simulink model "SF029A_StabyCmp"  (R2013b)
settings: Solver=FixedStepDiscrete  SolverMode=SingleTasking  StartTime=0.0  StopTime=1  FixedStep=0.002  RelTol=1e-3
values from neighbouring files (symbols this model uses):
  ARCHGLBPRM_2MILLISEC_SEC_F32 = DataDict.Constant    [SF029A_StabyCmp_DataDict.m]
  CMPINPLIM_MOTNWTMTR_F32 = DataDict.Constant    [SF029A_StabyCmp_DataDict.m]
  FLTINJ_STABYCMP_ASSICMD = DataDict.Constant    [SF029A_StabyCmp_DataDict.m]
undefined symbols (not defined in the file): StabyCmpNotchFil1Struct, StabyCmpNotchFil2Struct, StabyCmpNotchFil3Struct, StabyCmpNotchFil4Struct
libraries: NxtrMath x5, FixdToFloat x5, FloatToFixd x5, BilnrIntrpnMplX x4, Fil x2, NxtrLim x2, simulink x1, NxtrAbslt x1, LnrIntrpn x1
(part 1 of 2)
Description:
  | This function provides in-vehicle stability of EPS behavior.  To maximize steering feel, the function blends between two
  |  different tunings based on vehicle speed and low frequency handwheel torque.  Because system gains may get multiplied by various
  |  scale factors, either from serial communications or from other software functions, this function provides a second blending
  |  feature.
  | 
  | Some vehicle programs require a secondary, or "systematic", calculation of stability compensation followed by a correlation check.  The
  | systematic calculations usually must reside in a separate Memory Partition Unit (MPU), and switching between MPUs negatively impacts
  | system throughput.  This model is designed using the best-known implementation at this time.
settings Model: Creator=lzz0tm  LastModifiedBy=XZB1DB
settings Model: ModifiedHistory=|
  | 001
  | Initial release
  | K. Derry
  | n/a
  | 
  | 002
  | WHAT IS THIS ?????????????
  | 
  | 003
  | Move signal summation into SF-34 Assist Firewall.
  | Added AsstFW_Active as new input.
  | K. Derry
  | 19-Apr-2012
  | ICR-3358
  | 
  | 004
  | Addition of LPF of handwheel torque to the compensator blend tables.
  | Changed blend tables from 5x5 to 8x6 (speed x torq)
  | Price Lefler
  | 27-Jun-2012
  | ICR-3562
  | 
  | 005
  | Added functionality to allow compensators 2 and 4 to blend to zero (create two new calibrations)
  | Added 8.8Nm final saturation block to match code. (ref Anomaly 3559)
  | M. Hales
  | 24-Sep-2012
  | ICR-3754
  | Anom-3559
  | 
  | 006
  | Eliminate redundant compensator for BaseAssist input.
  | Eliminate output named BaseAssist_StCmp.
  | Add diverse Systematic Stability Comp.
  | Add correlation check and NTC output signal.
  | Reduce table sizes to 6 vehicle speeds, 5 points each.
  | Eliminate supplemental Word doc.
  | K. Derry
  | 12-Feb-2013
  | ICR-3950
  | 
  | 
  | 007
  | Add Pstep/Nstep counter to Correlation Check.
  | Change verbiage of v006 change log (did not eliminate 3-4 blend table).
  | Add simulation display variable to represent existing code's "StabilityComp2_SysAssistCmd" signal.
  | K. Derry
  | 15-Apr-2013
  | ICR-4078
settings SolverCC: AutoInsertRateTranBlk=on  InsertRTBMode=Always
settings DataIOCC: LimitDataPoints=off  SaveFormat=Structure  ReturnWorkspaceOutputs=on
settings OptimizationCC: BlockReduction=off  InlineParams=on  ZeroExternalMemoryAtStartup=off  ZeroInternalMemoryAtStartup=off  OptimizeModelRefInitCode=on  LifeSpan=1
settings DebuggingCC: ConsistencyChecking=warning  ArrayBoundsChecking=warning  SignalInfNanChecking=error  SignalRangeChecking=warning  UnderspecifiedInitializationDetection=Simplified  SolverPrmCheckMsg=error  InheritedTsInSrcMsg=error  DiscreteInheritContinuousMsg=error  SingleTaskRateTransMsg=error  TasksWithSamePriorityMsg=error  SigSpecEnsureSampleTimeMsg=error  CheckMatrixSingularityMsg=error  ParameterUnderflowMsg=error  ParameterPrecisionLossMsg=error  ParameterTunabilityLossMsg=error  FixptConstUnderflowMsg=warning  FixptConstOverflowMsg=warning  VectorMatrixConversionMsg=error  SignalLabelMismatchMsg=error  UnconnectedInputMsg=error  UnconnectedOutputMsg=error  UnconnectedLineMsg=error  SFcnCompatibilityMsg=error  UniqueDataStoreMsg=warning  BusObjectLabelMismatch=error  RootOutportRequireBusObject=error  AssertControl=DisableAll  ModelReferenceIOMsg=error  ModelReferenceVersionMismatchMessage=warning  ModelReferenceIOMismatchMessage=error  ModelReferenceCSMismatchMessage=warning  ModelReferenceDataLoggingMessage=error  StateNameClashWarn=warning  StrictBusMsg=ErrorOnBusTreatedAsVector  NonBusSignalsTreatedAsBus=error  SFUnexpectedBacktrackingDiag=error  SFInvalidInputDataAccessInChartInitDiag=error  SFNoUnconditionalDefaultTransitionDiag=error  SFTransitionOutsideNaturalParentDiag=error  SFUnconditionalTransitionShadowingDiag=error  SFUndirectedBroadcastEventsDiag=error
settings ModelReferenceCC: ModelReferenceNumInstancesAllowed=Single
settings RTWCC: SystemTargetFile=autosar.tlc  GenCodeOnly=on  TemplateMakefile=ert_default_tmf  Description=AUTOSAR  GenerateReport=on  ProcessScript=autosar_make_rtw_hook  LaunchReport=on
settings CodeAppCC: GenerateComments=off  IgnoreCustomStorageClasses=off  CustomSymbolStrType=$N$R$M  CustomSymbolStrBlkIO=$N$M  SimulinkBlockComments=off
settings STFCustomTargetCC: ParMdlRefBuildCompliant=on  CompOptLevelCompliant=on  IncludeMdlTerminateFcn=off  CombineOutputUpdateFcns=on  SuppressErrorStatus=on  ERTFirstTimeCompliant=on  ERTCustomFileBanners=on  SupportNonFinite=off  SupportComplex=off  SupportContinuousTime=off  SupportNonInlinedSFcns=off  MATLABClassNameForMDSCustomization=Simulink.SoftwareTarget.ERTCustomization  AutosarCompliant=on  GRTInterface=off  SystemTargetFile=autosar.tlc
settings ERTTargetCC: CodeReplacementLibrary=ANSI_C  ConcurrentExecutionCompliant=off  IncludeMdlTerminateFcn=off  SuppressErrorStatus=on  SupportNonFinite=off  SupportComplex=off  ModelStepFunctionPrototypeControlCompliant=off  CPPClassGenCompliant=off  AutosarCompliant=on  InlinedParameterPlacement=NonHierarchical  ERTCustomFileTemplate=example_file_process.tlc  EnableUserReplacementTypes=on

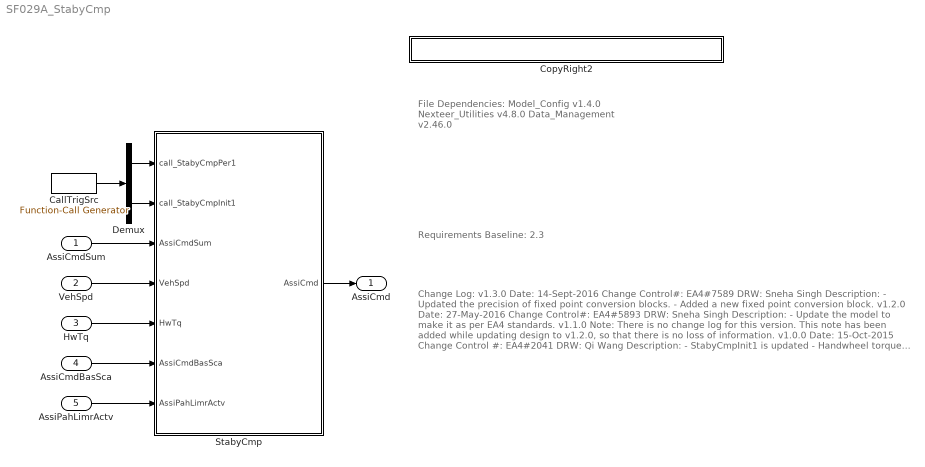
== system SF029A_StabyCmp ==
  note: File Dependencies:
      |
      | Model_Config v1.4.0
      | Nexteer_Utilities v4.8.0
      | Data_Management v2.46.0
  note: Requirements Baseline: 2.3
  note: Change Log:
      |
      | v1.3.0
      | Date: 14-Sept-2016
      | Change Control#: EA4#7589
      | DRW: Sneha Singh
      | Description:
      | - Updated the precision of fixed point conversion blocks.
      | - Added a new fixed point conversion block.
      |
      | v1.2.0
      | Date: 27-May-2016
      | Change Control#: EA4#5893
      | DRW: Sneha Singh
      | Description:
      | - Update the model to make it as per EA4 standards.
      |
      | v1.1.0
      | Note: There is no change log for this version. This note has been
      | added while updating design to v1.2.0, so that there is no loss of
      | information.
      |
      | v1.0.0
      | Date: 15-Oct-2015
      | Change Control #: EA4#2041
      | DRW:  Qi Wang
      | Description:
      | - StabyCmpInit1 is updated
      | - Handwheel torque Low-Pass filter is updated based on 2015 FDD standard
      | - PIMs are updated in the model
  AssiCmdSum : Inport  RequirementInfo="{'linktype_rmi_doors' '0000a537 (/E-STEER Core/SubSystem Specifications/Application Functions/SF029A Stability Compensation)' '#SF029A_70' 'true' 'REQ:  SF029A_70' '' } %GIDa_565dcead_0bc7_40e5_b597_0c44695b6e32"
  VehSpd : Inport  RequirementInfo="{'linktype_rmi_doors' '0000a537 (/E-STEER Core/SubSystem Specifications/Application Functions/SF029A Stability Compensation)' '#SF029A_71' 'true' 'REQ:  SF029A_71' '' } %GIDa_d041abf9_c003_46d5_8c18_c9951e1c5ae1"  Port=2
  HwTq : Inport  RequirementInfo="{'linktype_rmi_doors' '0000a537 (/E-STEER Core/SubSystem Specifications/Application Functions/SF029A Stability Compensation)' '#SF029A_72' 'true' 'REQ:  SF029A_72' '' } %GIDa_dac3164c_f505_4145_8387_4495c6482d18"  Port=3
  AssiCmdBasSca : Inport  RequirementInfo="{'linktype_rmi_doors' '0000a537 (/E-STEER Core/SubSystem Specifications/Application Functions/SF029A Stability Compensation)' '#SF029A_73' 'true' 'REQ:  SF029A_73' '' } %GIDa_6f59ef3f_1a47_4437_bb00_97dd4e07e97c"  Port=4
  AssiPahLimrActv : Inport  RequirementInfo="{'linktype_rmi_doors' '0000a537 (/E-STEER Core/SubSystem Specifications/Application Functions/SF029A Stability Compensation)' '#SF029A_74' 'true' 'REQ:  SF029A_74' '' } %GIDa_e47b1a13_d7c8_4723_b64a_afff46581b7f"  Port=5
  CallTrigSrc : simulink/Ports & Subsystems/Function-Call Generator  RequirementInfo={} %GIDa_050e24ca_7982_42dd_bdc0_09948903a5d2  sample_time=0.004  numberOfIterations=1
  CopyRight2 : Subsystem  Description=|  mask(Copyright Information){none=on}
      | Copyright info block.                                               
      |                                                                     
      | Place copyright information at the top of every subsystem in design.
      mask prompts: none "No parameters"
      mask help: Place copyright information at the top of every subsystem in design.
      mask Display:
      | NxtrConf = 'Nexteer Confidential';
      | 
      | sys = bdroot; %handle for the current model ("system")
      | first = get_param(sys,'Created');
      | if(isempty(first))
      |     first = datestr(now,'yyyy');
      | else
      |     first = first(end-3:end);  %year is last four digits
      | end
      | 
      | last = get_param(sys,'LastModifiedDate');
      | if isempty(last)
      |     last = datestr(now,'yyyy');
      | else
      |     last = last(end-3:end);
      | end
      | 
      | if strcmp(first,last)
      |     fprintf('%s -- Copyright %s Nexteer',NxtrConf,first)
      | else
      |     fprintf('%s -- %s%s- %s Nexteer',NxtrConf,char(169),first,last)
      | end
  Demux : Demux  Outputs=2
  StabyCmp : Subsystem
  AssiCmd : Outport  RequirementInfo="{'linktype_rmi_doors' '0000a537 (/E-STEER Core/SubSystem Specifications/Application Functions/SF029A Stability Compensation)' '#SF029A_76' 'true' 'REQ:  SF029A_76' '' ; 'linktype_rmi_doors' '0000a537 (/E-STEER Core/SubSystem Specifications/Application Functions/SF029A Stability Compensation)' '#SF029A_99' 'true' 'REQ:  SF029A_99' '' ; 'linktype_rmi_doors' '0000a537 (/E-STEER Core/SubSystem Specifications/Application Functions/SF029A Stability Compensation)' '#SF029A_101' 'true' 'REQ:  SF029A_101' '' } %GIDa_32d67de0_2e1d_41c7_bc59_3e04764ffb88"
  wires:
  StabyCmp/1(AssiCmd) -> AssiCmd/1
  AssiCmdSum/1 -> StabyCmp/3(AssiCmdSum)
  VehSpd/1 -> StabyCmp/4(VehSpd)
  HwTq/1 -> StabyCmp/5(HwTq)
  AssiCmdBasSca/1 -> StabyCmp/6(AssiCmdBasSca)
  AssiPahLimrActv/1 -> StabyCmp/7(AssiPahLimrActv)
  Demux/1 -> StabyCmp/1(call_StabyCmpPer1)
  Demux/2 -> StabyCmp/2(call_StabyCmpInit1)
  CallTrigSrc/1 -> Demux/1

== system SF029A_StabyCmp/CopyRight2 ==

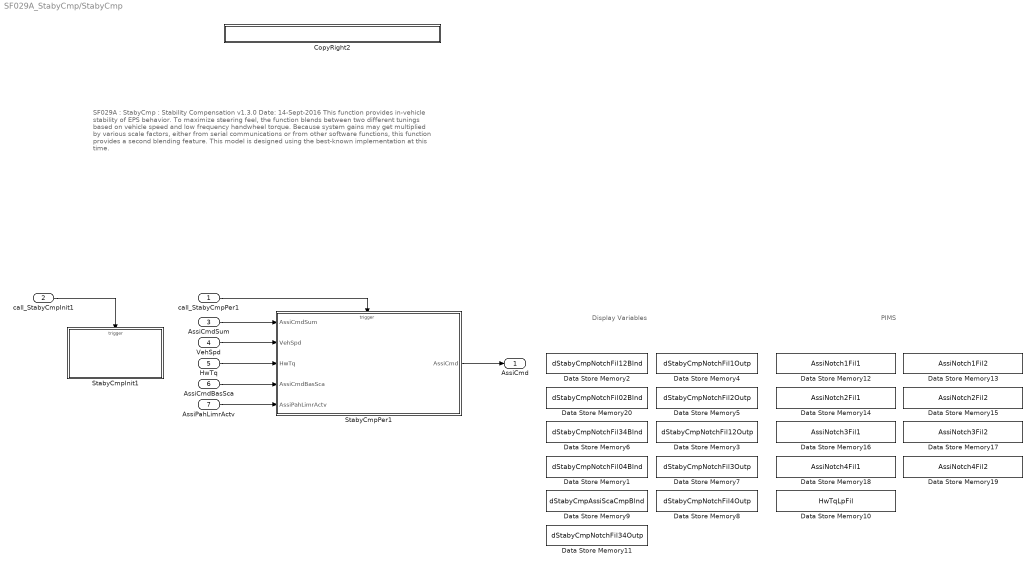
== system SF029A_StabyCmp/StabyCmp ==
  note: SF029A : StabyCmp : Stability Compensation
      | v1.3.0
      | Date: 14-Sept-2016
      |
      |
      |   This function provides in-vehicle stability of EPS behavior. To maximize steering feel,
      |   the function blends between two different tunings based on vehicle speed and low frequency
      |   handwheel torque. Because system gains may get multiplied by various scale factors, either
      |   from serial communications or from other software functions, this function provides a second blending feature.
      |   This model is designed using the best-known implementation at this time.
  note: Display Variables
  note: PIMS
  call_StabyCmpPer1 : Inport
  call_StabyCmpInit1 : Inport  Port=2
  AssiCmdSum : Inport  Port=3
  VehSpd : Inport  Port=4
  HwTq : Inport  Port=5
  AssiCmdBasSca : Inport  Port=6
  AssiPahLimrActv : Inport  Port=7
  CopyRight2 : Subsystem  Description=|  mask(Copyright Information){none=on}
      | Copyright info block.                                               
      |                                                                     
      | Place copyright information at the top of every subsystem in design.
      mask prompts: none "No parameters"
      mask help: Place copyright information at the top of every subsystem in design.
      mask Display:
      | NxtrConf = 'Nexteer Confidential';
      | 
      | sys = bdroot; %handle for the current model ("system")
      | first = get_param(sys,'Created');
      | if(isempty(first))
      |     first = datestr(now,'yyyy');
      | else
      |     first = first(end-3:end);  %year is last four digits
      | end
      | 
      | last = get_param(sys,'LastModifiedDate');
      | if isempty(last)
      |     last = datestr(now,'yyyy');
      | else
      |     last = last(end-3:end);
      | end
      | 
      | if strcmp(first,last)
      |     fprintf('%s -- Copyright %s Nexteer',NxtrConf,first)
      | else
      |     fprintf('%s -- %s%s- %s Nexteer',NxtrConf,char(169),first,last)
      | end
  Data Store Memory1 : DataStoreMemory  DataStoreName=dStabyCmpNotchFil04Blnd  ReadBeforeWriteMsg=warning  WriteAfterWriteMsg=warning  WriteAfterReadMsg=warning  StateMustResolveToSignalObject=on
  Data Store Memory10 : DataStoreMemory  DataStoreName=HwTqLpFil  InitialValue=[]  StateMustResolveToSignalObject=on
  Data Store Memory11 : DataStoreMemory  DataStoreName=dStabyCmpNotchFil34Outp  ReadBeforeWriteMsg=warning  WriteAfterWriteMsg=warning  WriteAfterReadMsg=warning  StateMustResolveToSignalObject=on
  Data Store Memory12 : DataStoreMemory  DataStoreName=AssiNotch1Fil1  StateMustResolveToSignalObject=on
  Data Store Memory13 : DataStoreMemory  DataStoreName=AssiNotch1Fil2  InitialValue=[]  StateMustResolveToSignalObject=on
  Data Store Memory14 : DataStoreMemory  DataStoreName=AssiNotch2Fil1  InitialValue=[]  StateMustResolveToSignalObject=on
  Data Store Memory15 : DataStoreMemory  DataStoreName=AssiNotch2Fil2  InitialValue=[]  StateMustResolveToSignalObject=on
  Data Store Memory16 : DataStoreMemory  DataStoreName=AssiNotch3Fil1  InitialValue=[]  StateMustResolveToSignalObject=on
  Data Store Memory17 : DataStoreMemory  DataStoreName=AssiNotch3Fil2  InitialValue=[]  StateMustResolveToSignalObject=on
  Data Store Memory18 : DataStoreMemory  DataStoreName=AssiNotch4Fil1  InitialValue=[]  StateMustResolveToSignalObject=on
  Data Store Memory19 : DataStoreMemory  DataStoreName=AssiNotch4Fil2  InitialValue=[]  StateMustResolveToSignalObject=on
  Data Store Memory2 : DataStoreMemory  DataStoreName=dStabyCmpNotchFil12Blnd  ReadBeforeWriteMsg=warning  WriteAfterWriteMsg=warning  WriteAfterReadMsg=warning  StateMustResolveToSignalObject=on
  Data Store Memory20 : DataStoreMemory  DataStoreName=dStabyCmpNotchFil02Blnd  ReadBeforeWriteMsg=warning  WriteAfterWriteMsg=warning  WriteAfterReadMsg=warning  StateMustResolveToSignalObject=on
  Data Store Memory3 : DataStoreMemory  DataStoreName=dStabyCmpNotchFil12Outp  ReadBeforeWriteMsg=warning  WriteAfterWriteMsg=warning  WriteAfterReadMsg=warning  StateMustResolveToSignalObject=on
  Data Store Memory4 : DataStoreMemory  DataStoreName=dStabyCmpNotchFil1Outp  ReadBeforeWriteMsg=warning  WriteAfterWriteMsg=warning  WriteAfterReadMsg=warning  StateMustResolveToSignalObject=on
  Data Store Memory5 : DataStoreMemory  DataStoreName=dStabyCmpNotchFil2Outp  ReadBeforeWriteMsg=warning  WriteAfterWriteMsg=warning  WriteAfterReadMsg=warning  StateMustResolveToSignalObject=on
  Data Store Memory6 : DataStoreMemory  DataStoreName=dStabyCmpNotchFil34Blnd  ReadBeforeWriteMsg=warning  WriteAfterWriteMsg=warning  WriteAfterReadMsg=warning  StateMustResolveToSignalObject=on
  Data Store Memory7 : DataStoreMemory  DataStoreName=dStabyCmpNotchFil3Outp  ReadBeforeWriteMsg=warning  WriteAfterWriteMsg=warning  WriteAfterReadMsg=warning  StateMustResolveToSignalObject=on
  Data Store Memory8 : DataStoreMemory  DataStoreName=dStabyCmpNotchFil4Outp  ReadBeforeWriteMsg=warning  WriteAfterWriteMsg=warning  WriteAfterReadMsg=warning  StateMustResolveToSignalObject=on
  Data Store Memory9 : DataStoreMemory  DataStoreName=dStabyCmpAssiScaCmpBlnd  ReadBeforeWriteMsg=warning  WriteAfterWriteMsg=warning  WriteAfterReadMsg=warning  StateMustResolveToSignalObject=on
  StabyCmpInit1 : Subsystem
  StabyCmpPer1 : Subsystem
  AssiCmd : Outport
  wires:
  AssiCmdSum/1 -> StabyCmpPer1/1(AssiCmdSum)
  VehSpd/1 -> StabyCmpPer1/2(VehSpd)
  HwTq/1 -> StabyCmpPer1/3(HwTq)
  AssiCmdBasSca/1 -> StabyCmpPer1/4(AssiCmdBasSca)
  AssiPahLimrActv/1 -> StabyCmpPer1/5(AssiPahLimrActv)
  StabyCmpPer1/1(AssiCmd) -> AssiCmd/1
  call_StabyCmpPer1/1 -> StabyCmpPer1/Trigger
  call_StabyCmpInit1/1 -> StabyCmpInit1/Trigger

== system SF029A_StabyCmp/StabyCmp/CopyRight2 ==

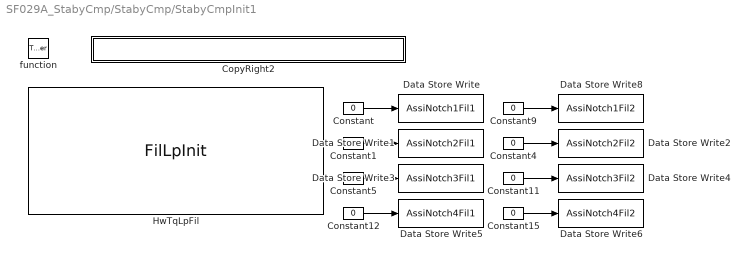
== system SF029A_StabyCmp/StabyCmp/StabyCmpInit1 ==
  function : TriggerPort  TriggerType=function-call
  Constant{,1,4..5,9,11..12,15} (8 alike) : Constant  Value=0  OutDataTypeStr=Inherit: Inherit via back propagation  SampleTime=-1
  CopyRight2 : Subsystem  Description=|  mask(Copyright Information){none=on}
      | Copyright info block.                                               
      |                                                                     
      | Place copyright information at the top of every subsystem in design.
      mask prompts: none "No parameters"
      mask help: Place copyright information at the top of every subsystem in design.
      mask Display:
      | NxtrConf = 'Nexteer Confidential';
      | 
      | sys = bdroot; %handle for the current model ("system")
      | first = get_param(sys,'Created');
      | if(isempty(first))
      |     first = datestr(now,'yyyy');
      | else
      |     first = first(end-3:end);  %year is last four digits
      | end
      | 
      | last = get_param(sys,'LastModifiedDate');
      | if isempty(last)
      |     last = datestr(now,'yyyy');
      | else
      |     last = last(end-3:end);
      | end
      | 
      | if strcmp(first,last)
      |     fprintf('%s -- Copyright %s Nexteer',NxtrConf,first)
      | else
      |     fprintf('%s -- %s%s- %s Nexteer',NxtrConf,char(169),first,last)
      | end
  Data Store Write : DataStoreWrite  DataStoreName=AssiNotch1Fil1  DataStoreElements=AssiNotch1Fil1
  Data Store Write1 : DataStoreWrite  DataStoreName=AssiNotch2Fil1  DataStoreElements=AssiNotch2Fil1
  Data Store Write2 : DataStoreWrite  DataStoreName=AssiNotch2Fil2  DataStoreElements=AssiNotch2Fil2
  Data Store Write3 : DataStoreWrite  DataStoreName=AssiNotch3Fil1  DataStoreElements=AssiNotch3Fil1
  Data Store Write4 : DataStoreWrite  DataStoreName=AssiNotch3Fil2  DataStoreElements=AssiNotch3Fil2
  Data Store Write5 : DataStoreWrite  DataStoreName=AssiNotch4Fil1  DataStoreElements=AssiNotch4Fil1
  Data Store Write6 : DataStoreWrite  DataStoreName=AssiNotch4Fil2  DataStoreElements=AssiNotch4Fil2
  Data Store Write8 : DataStoreWrite  DataStoreName=AssiNotch1Fil2  DataStoreElements=AssiNotch1Fil2
  HwTqLpFil : Fil/FilLpInit  Ic=0  Ts=ARCHGLBPRM_2MILLISEC_SEC_F32  Freq=StabyCmpHwTqLpFilFrq  StVar=HwTqLpFil
  wires:
  Constant/1 -> Data Store Write/1
  Constant9/1 -> Data Store Write8/1
  Constant1/1 -> Data Store Write1/1
  Constant4/1 -> Data Store Write2/1
  Constant5/1 -> Data Store Write3/1
  Constant11/1 -> Data Store Write4/1
  Constant12/1 -> Data Store Write5/1
  Constant15/1 -> Data Store Write6/1

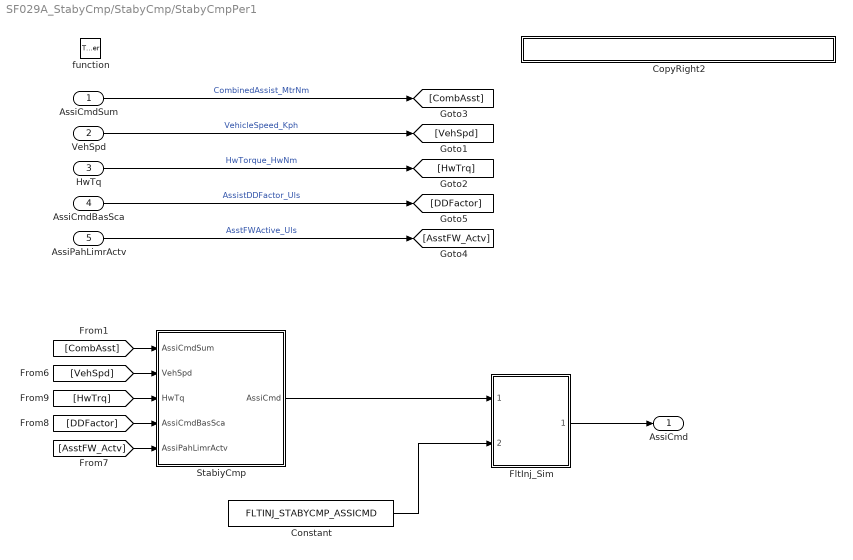
== system SF029A_StabyCmp/StabyCmp/StabyCmpPer1 ==
  AssiCmdSum : Inport
  VehSpd : Inport  Port=2
  HwTq : Inport  Port=3
  AssiCmdBasSca : Inport  Port=4
  AssiPahLimrActv : Inport  Port=5
  function : TriggerPort  TriggerType=function-call  PortDimensions=1
  Constant : Constant  Value=FLTINJ_STABYCMP_ASSICMD
  CopyRight2 : Subsystem  Description=|  mask(Copyright Information){none=on}
      | Copyright info block.                                               
      |                                                                     
      | Place copyright information at the top of every subsystem in design.
      mask prompts: none "No parameters"
      mask help: Place copyright information at the top of every subsystem in design.
      mask Display:
      | NxtrConf = 'Nexteer Confidential';
      | 
      | sys = bdroot; %handle for the current model ("system")
      | first = get_param(sys,'Created');
      | if(isempty(first))
      |     first = datestr(now,'yyyy');
      | else
      |     first = first(end-3:end);  %year is last four digits
      | end
      | 
      | last = get_param(sys,'LastModifiedDate');
      | if isempty(last)
      |     last = datestr(now,'yyyy');
      | else
      |     last = last(end-3:end);
      | end
      | 
      | if strcmp(first,last)
      |     fprintf('%s -- Copyright %s Nexteer',NxtrConf,first)
      | else
      |     fprintf('%s -- %s%s- %s Nexteer',NxtrConf,char(169),first,last)
      | end
  FltInj_Sim : Subsystem  RequirementInfo="{'linktype_rmi_doors' '0000a537 (/E-STEER Core/SubSystem Specifications/Application Functions/SF029A Stability Compensation)' '#SF029A_106' 'true' 'REQ:  SF029A_106' '' } %GIDa_4f586a3b_dea5_4a76_a847_596b049200d7"  TreatAsAtomicUnit=on  VariantControl=FltInj_sim  mask(Fault_Injection){}
      mask help: Fault Injection is a simulation only block for EA3 and EA4 programs.
  StabiyCmp : Subsystem
  AssiCmd : Outport
  wires:
  VehSpd/1 -> [VehSpd]  "VehicleSpeed_Kph"
  HwTq/1 -> [HwTrq]  "HwTorque_HwNm"
  [CombAsst] -> StabiyCmp/1(AssiCmdSum)
  [VehSpd] -> StabiyCmp/2(VehSpd)
  [HwTrq] -> StabiyCmp/3(HwTq)
  [DDFactor] -> StabiyCmp/4(AssiCmdBasSca)
  AssiCmdSum/1 -> [CombAsst]  "CombinedAssist_MtrNm"
  AssiCmdBasSca/1 -> [DDFactor]  "AssistDDFactor_Uls"
  AssiPahLimrActv/1 -> [AsstFW_Actv]  "AsstFWActive_Uls"
  [AsstFW_Actv] -> StabiyCmp/5(AssiPahLimrActv)
  Constant/1 -> FltInj_Sim/2(FltInjCon)
  FltInj_Sim/1(AssiCmd) -> AssiCmd/1
  StabiyCmp/1(AssiCmd) -> FltInj_Sim/1(AssiCmdOutp)

== system SF029A_StabyCmp/StabyCmp/StabyCmpInit1/CopyRight2 ==

== system SF029A_StabyCmp/StabyCmp/StabyCmpPer1/CopyRight2 ==

== system SF029A_StabyCmp/StabyCmp/StabyCmpPer1/FltInj_Sim ==
  note: This block requires no modification by FDD author.
      |
      | This block does not actually simulate any fault injection.  It is simply a pass-thru.
      |
      | The port (#2) simply terminates its signal, but we are trying to force the FDD author
      | to properly use the Constant in FDD model.
  note: EA4.x Fault Injection
  note: Inport #2 must be Constant
  AssiCmdOutp : Inport
  FltInjCon : Inport  Port=2
  CopyRight2 : Subsystem  Description=|  mask(Copyright Information){none=on}
      | Copyright info block.                                               
      |                                                                     
      | Place copyright information at the top of every subsystem in design.
      mask prompts: none "No parameters"
      mask help: Place copyright information at the top of every subsystem in design.
      mask Display:
      | NxtrConf = 'Nexteer Confidential';
      | 
      | sys = bdroot; %handle for the current model ("system")
      | first = get_param(sys,'Created');
      | if(isempty(first))
      |     first = datestr(now,'yyyy');
      | else
      |     first = first(end-3:end);  %year is last four digits
      | end
      | 
      | last = get_param(sys,'LastModifiedDate');
      | if isempty(last)
      |     last = datestr(now,'yyyy');
      | else
      |     last = last(end-3:end);
      | end
      | 
      | if strcmp(first,last)
      |     fprintf('%s -- Copyright %s Nexteer',NxtrConf,first)
      | else
      |     fprintf('%s -- %s%s- %s Nexteer',NxtrConf,char(169),first,last)
      | end
  Terminator : Terminator
  AssiCmd : Outport
  wires:
  AssiCmdOutp/1 -> AssiCmd/1
  FltInjCon/1 -> Terminator/1

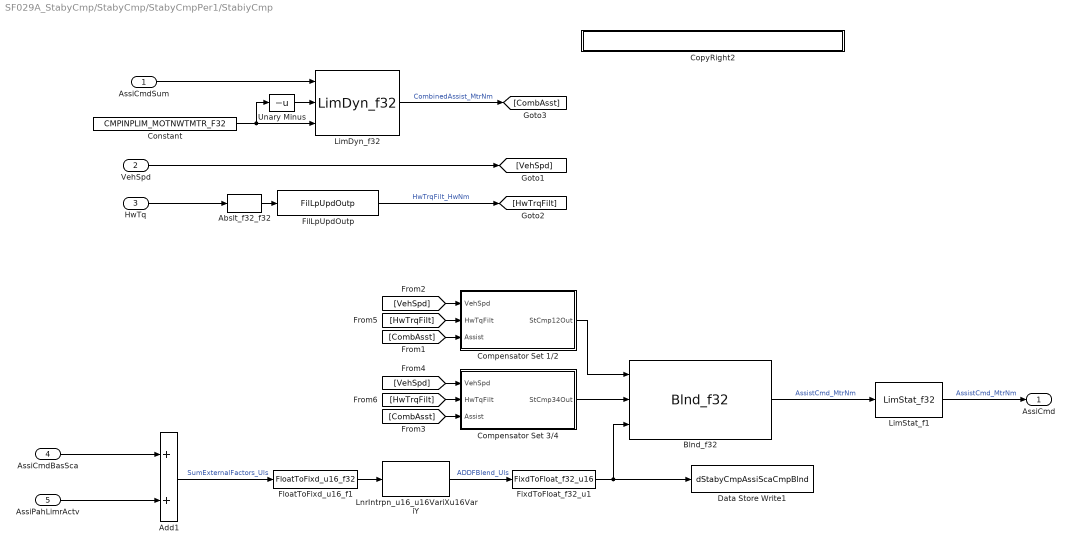
== system SF029A_StabyCmp/StabyCmp/StabyCmpPer1/StabiyCmp ==
  AssiCmdSum : Inport
  VehSpd : Inport  Port=2
  HwTq : Inport  Port=3
  AssiCmdBasSca : Inport  RequirementInfo="{'linktype_rmi_doors' '0000a537 (/E-STEER Core/SubSystem Specifications/Application Functions/SF029A Stability Compensation)' '#SF029A_93' 'true' 'REQ:  SF029A_93' '' } %GIDa_e52f2ad1_fd47_421d_8c08_8c30a1c05406"  Port=4
      settings: AttributesFormatString=%<Tag>
  AssiPahLimrActv : Inport  RequirementInfo="{'linktype_rmi_doors' '0000a537 (/E-STEER Core/SubSystem Specifications/Application Functions/SF029A Stability Compensation)' '#SF029A_93' 'true' 'REQ:  SF029A_93' '' } %GIDa_1d5b88ab_396b_4d89_9700_00f5ed32e8aa"  Port=5
      settings: AttributesFormatString=%<Tag>
  Abslt_f32_f32 : NxtrAbslt/Abslt_f32_f32  RequirementInfo="{'linktype_rmi_doors' '0000a537 (/E-STEER Core/SubSystem Specifications/Application Functions/SF029A Stability Compensation)' '#SF029A_80' 'true' 'REQ:  SF029A_80' '' } %GIDa_e58e449f_99f0_42c1_896c_b4bed6e53470"  SFunctionSpec=single y1 = Abslt_f32_f32(single u1)
      settings: AttributesFormatString=%<Name>
  Add1 : Sum  RequirementInfo="{'linktype_rmi_doors' '0000a537 (/E-STEER Core/SubSystem Specifications/Application Functions/SF029A Stability Compensation)' '#SF029A_93' 'true' 'REQ:  SF029A_93' '' } %GIDa_2f792d03_7f63_496e_bb4b_c1c151e55f4e"
      settings: AttributesFormatString=%<Tag>
  Blnd_f32 : NxtrMath/Blnd_f32  RequirementInfo="{'linktype_rmi_doors' '0000a537 (/E-STEER Core/SubSystem Specifications/Application Functions/SF029A Stability Compensation)' '#SF029A_93' 'true' 'REQ:  SF029A_93' '' } %GIDa_aac33a22_20b9_4488_865f_8251dad173fa"  SFunctionSpec=single y1 = Blnd_f32(single u1, single u2, single u3)  Parameter3=on
      settings: AttributesFormatString=%<Name>
  Compensator Set 1/2 : Subsystem
  Compensator Set 3/4 : Subsystem
  Constant : Constant  RequirementInfo="{'linktype_rmi_doors' '0000a537 (/E-STEER Core/SubSystem Specifications/Application Functions/SF029A Stability Compensation)' '#SF029A_81' 'true' 'REQ:  SF029A_81' '' } %GIDa_0fa329a0_f831_46cf_b20c_4e9a4dd8937d"  Value=CMPINPLIM_MOTNWTMTR_F32
  CopyRight2 : Subsystem  Description=|  mask(Copyright Information){none=on}
      | Copyright info block.                                               
      |                                                                     
      | Place copyright information at the top of every subsystem in design.
      mask prompts: none "No parameters"
      mask help: Place copyright information at the top of every subsystem in design.
      mask Display:
      | NxtrConf = 'Nexteer Confidential';
      | 
      | sys = bdroot; %handle for the current model ("system")
      | first = get_param(sys,'Created');
      | if(isempty(first))
      |     first = datestr(now,'yyyy');
      | else
      |     first = first(end-3:end);  %year is last four digits
      | end
      | 
      | last = get_param(sys,'LastModifiedDate');
      | if isempty(last)
      |     last = datestr(now,'yyyy');
      | else
      |     last = last(end-3:end);
      | end
      | 
      | if strcmp(first,last)
      |     fprintf('%s -- Copyright %s Nexteer',NxtrConf,first)
      | else
      |     fprintf('%s -- %s%s- %s Nexteer',NxtrConf,char(169),first,last)
      | end
  Data Store Write1 : DataStoreWrite  DataStoreName=dStabyCmpAssiScaCmpBlnd
  FilLpUpdOutp : Fil/FilLpUpdOutp  RequirementInfo="{'linktype_rmi_doors' '0000a537 (/E-STEER Core/SubSystem Specifications/Application Functions/SF029A Stability Compensation)' '#SF029A_80' 'true' 'REQ:  SF029A_80' '' } %GIDa_e50dfd97_808a_4ecb_9afb_8d1ce7d9c01b"  StVar=HwTqLpFil
      settings: AttributesFormatString=StVar: %<StVar>
  FixdToFloat_f32_u1 : FixdToFloat/FixdToFloat_f32_u16  RequirementInfo="{'linktype_rmi_doors' '0000a537 (/E-STEER Core/SubSystem Specifications/Application Functions/SF029A Stability Compensation)' '#SF029A_93' 'true' 'REQ:  SF029A_93' '' } %GIDa_8db98107_d72d_46ce_bb11_b21278a91118"  Param1=14
  FloatToFixd_u16_f1 : FloatToFixd/FloatToFixd_u16_f32  Param1=14
  LimDyn_f32 : NxtrLim/LimDyn_f32  RequirementInfo="{'linktype_rmi_doors' '0000a537 (/E-STEER Core/SubSystem Specifications/Application Functions/SF029A Stability Compensation)' '#SF029A_81' 'true' 'REQ:  SF029A_81' '' } %GIDa_138aed1d_98dc_4852_adea_0252395672f7"
  LimStat_f1 : NxtrLim/LimStat_f32  RequirementInfo="{'linktype_rmi_doors' '0000a537 (/E-STEER Core/SubSystem Specifications/Application Functions/SF029A Stability Compensation)' '#SF029A_94' 'true' 'REQ:  SF029A_94' '' } %GIDa_e5042578_7661_4cd7_b5a9_512a3779a978"  LoLim=SYSGLBPRM_MOTTQCMDLOLIM_MOTNWTMTR_F32  HiLim=SYSGLBPRM_MOTTQCMDHILIM_MOTNWTMTR_F32
      settings: AttributesFormatString=|
      | Low Limit: %<LoLim>
      | High Limit:%<HiLim>
  LnrIntrpn_u16_u16VariXu16VariY : LnrIntrpn/LnrIntrpn_u16_u16VariXu16VariY  RequirementInfo="{'linktype_rmi_doors' '0000a537 (/E-STEER Core/SubSystem Specifications/Application Functions/SF029A Stability Compensation)' '#SF029A_93' 'true' 'REQ:  SF029A_93' '' } %GIDa_788cf387_8266_4e90_8950_327c02d399c2"  XTbl=StabyCmpAssiScaBlndX  YTbl=StabyCmpAssiScaBlndY
      settings: AttributesFormatString=|
      | Lnr ( u16VariX , u16VariY )
      | XTbl: %<XTbl>
      | YTbl: %<YTbl>
  Unary Minus : UnaryMinus  RequirementInfo="{'linktype_rmi_doors' '0000a537 (/E-STEER Core/SubSystem Specifications/Application Functions/SF029A Stability Compensation)' '#SF029A_81' 'true' 'REQ:  SF029A_81' '' } %GIDa_4787fd09_3b48_441a_baf7_bf2ffd79fe3e"
  AssiCmd : Outport
  wires:
  Compensator Set 3/4/1(StCmp34Out) -> Blnd_f32/2
  Compensator Set 1/2/1(StCmp12Out) -> Blnd_f32/1
  Blnd_f32/1 -> LimStat_f1/1  "AssistCmd_MtrNm"
  VehSpd/1 -> [VehSpd]
  AssiCmdSum/1 -> LimDyn_f32/1
  Add1/1 -> FloatToFixd_u16_f1/1  "SumExternalFactors_Uls"
  LnrIntrpn_u16_u16VariXu16VariY/1 -> FixdToFloat_f32_u1/1  "ADDFBlend_Uls"
  AssiCmdBasSca/1 -> Add1/1
  AssiPahLimrActv/1 -> Add1/2
  LimDyn_f32/1 -> [CombAsst]  "CombinedAssist_MtrNm"
  LimStat_f1/1 -> AssiCmd/1  "AssistCmd_MtrNm"
  [VehSpd] -> Compensator Set 1/2/1(VehSpd)
  [CombAsst] -> Compensator Set 1/2/3(Assist)
  Abslt_f32_f32/1 -> FilLpUpdOutp/1
  HwTq/1 -> Abslt_f32_f32/1
  FilLpUpdOutp/1 -> [HwTrqFilt]  "HwTrqFilt_HwNm"
  [HwTrqFilt] -> Compensator Set 1/2/2(HwTqFilt)
  [VehSpd] -> Compensator Set 3/4/1(VehSpd)
  [HwTrqFilt] -> Compensator Set 3/4/2(HwTqFilt)
  [CombAsst] -> Compensator Set 3/4/3(Assist)
  FixdToFloat_f32_u1/1 -> Blnd_f32/3, Data Store Write1/1
  Constant/1 -> Unary Minus/1, LimDyn_f32/3
  Unary Minus/1 -> LimDyn_f32/2
  FloatToFixd_u16_f1/1 -> LnrIntrpn_u16_u16VariXu16VariY/1

== system SF029A_StabyCmp/StabyCmp/StabyCmpPer1/FltInj_Sim/CopyRight2 ==

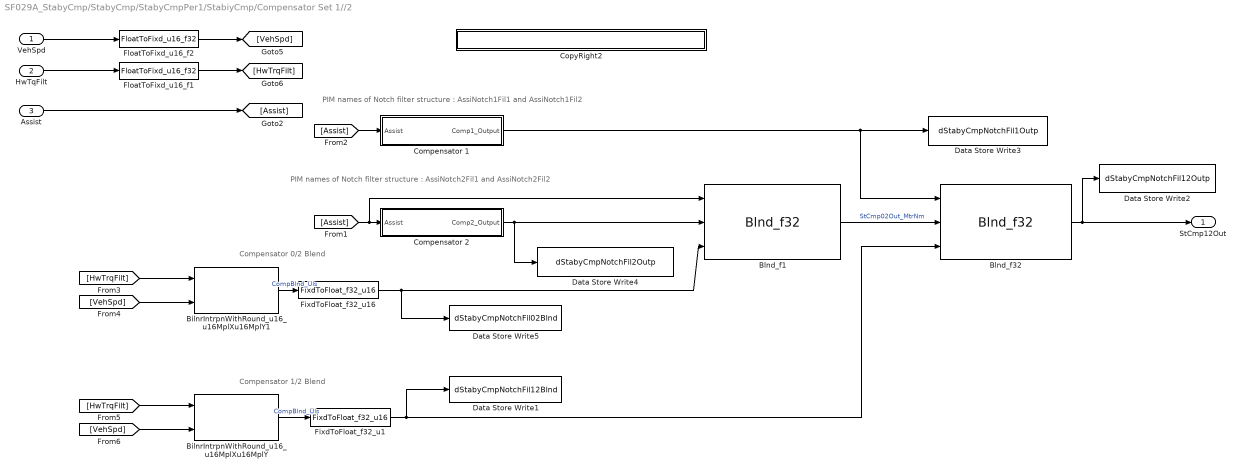
== system SF029A_StabyCmp/StabyCmp/StabyCmpPer1/StabiyCmp/Compensator Set 1//2 ==
  note: PIM names of Notch filter structure : AssiNotch1Fil1 and AssiNotch1Fil2
  note: Compensator 1/2 Blend
  note: Compensator 0/2 Blend
  note: PIM names of Notch filter structure : AssiNotch2Fil1 and AssiNotch2Fil2
  VehSpd : Inport
  HwTqFilt : Inport  Port=2
  Assist : Inport  Port=3
  BilnrIntrpnWithRound_u16_u16MplXu16MplY : BilnrIntrpnMplX/BilnrIntrpnWithRound_u16_u16MplXu16MplY  RequirementInfo="{'linktype_rmi_doors' '0000a537 (/E-STEER Core/SubSystem Specifications/Application Functions/SF029A Stability Compensation)' '#SF029A_86' 'true' 'REQ:  SF029A_86' '' } %GIDa_fadd72e6_d831_45ef_8099_953e3d2c1c69"  MplXTbl=StabyCmpNotchFilBlnd12TqX  MplYTbl=StabyCmpNotchFilBlnd12Y  BilnrSelnTbl=StabyCmpNotchFilBilnrBlndVehSpd
      settings: AttributesFormatString=|
      | Bilnr ( u16MplX , u16MplY )
      | XTbl: %<MplXTbl>
      | YTbl: %<MplYTbl>
      | BilnrSelnTbl: %<BilnrSelnTbl>
  BilnrIntrpnWithRound_u16_u16MplXu16MplY1 : BilnrIntrpnMplX/BilnrIntrpnWithRound_u16_u16MplXu16MplY  RequirementInfo="{'linktype_rmi_doors' '0000a537 (/E-STEER Core/SubSystem Specifications/Application Functions/SF029A Stability Compensation)' '#SF029A_85' 'true' 'REQ:  SF029A_85' '' } %GIDa_42ed8477_37e6_4b44_a66a_f9bae03e7c36"  MplXTbl=StabyCmpNotchFilBlnd12TqX  MplYTbl=StabyCmpNotchFilBlnd02Y  BilnrSelnTbl=StabyCmpNotchFilBilnrBlndVehSpd
      settings: AttributesFormatString=|
      | Bilnr ( u16MplX , u16MplY )
      | XTbl: %<MplXTbl>
      | YTbl: %<MplYTbl>
      | BilnrSelnTbl: %<BilnrSelnTbl>
  Blnd_f1 : NxtrMath/Blnd_f32  RequirementInfo="{'linktype_rmi_doors' '0000a537 (/E-STEER Core/SubSystem Specifications/Application Functions/SF029A Stability Compensation)' '#SF029A_85' 'true' 'REQ:  SF029A_85' '' } %GIDa_dba1abdf_517a_44f0_a412_df1ce507f594"  SFunctionSpec=single y1 = Blnd_f32(single u1, single u2, single u3)  Parameter3=on
      settings: AttributesFormatString=%<Name>
  Blnd_f32 : NxtrMath/Blnd_f32  RequirementInfo="{'linktype_rmi_doors' '0000a537 (/E-STEER Core/SubSystem Specifications/Application Functions/SF029A Stability Compensation)' '#SF029A_86' 'true' 'REQ:  SF029A_86' '' } %GIDa_db82eb3d_baf5_47e3_9dad_3db9927823cc"  SFunctionSpec=single y1 = Blnd_f32(single u1, single u2, single u3)  Parameter3=on
      settings: AttributesFormatString=%<Name>
  Compensator 1 : Subsystem  RequirementInfo="{'linktype_rmi_doors' '0000a537 (/E-STEER Core/SubSystem Specifications/Application Functions/SF029A Stability Compensation)' '#SF029A_84' 'true' 'REQ:  SF029A_84' '' ; 'linktype_rmi_doors' '0000a537 (/E-STEER Core/SubSystem Specifications/Application Functions/SF029A Stability Compensation)' '#SF029A_86' 'true' 'REQ:  SF029A_86' '' } %GIDa_51cc23fa_f620_4c31_99b0_c4f508588dc0"  mask{B0=StabyCmpNotchFil1Struct.FilGainB0, B1=StabyCmpNotchFil1Struct.FilGainB1, B2=StabyCmpNotchFil1Struct.FilGainB2, A1=StabyCmpNotchFil1Struct.FilGainA1, A2=StabyCmpNotchFil1Struct.FilGainA2}
      settings: AttributesFormatString=%<Tag>
  Compensator 2 : Subsystem  RequirementInfo="{'linktype_rmi_doors' '0000a537 (/E-STEER Core/SubSystem Specifications/Application Functions/SF029A Stability Compensation)' '#SF029A_83' 'true' 'REQ:  SF029A_83' '' ; 'linktype_rmi_doors' '0000a537 (/E-STEER Core/SubSystem Specifications/Application Functions/SF029A Stability Compensation)' '#SF029A_85' 'true' 'REQ:  SF029A_85' '' } %GIDa_3662596c_3573_4bcf_b246_b1e5ed52c886"  mask{B0=StabyCmpNotchFil2Struct.FilGainB0, B1=StabyCmpNotchFil2Struct.FilGainB1, B2=StabyCmpNotchFil2Struct.FilGainB2, A1=StabyCmpNotchFil2Struct.FilGainA1, A2=StabyCmpNotchFil2Struct.FilGainA2}
      settings: AttributesFormatString=%<Tag>
  CopyRight2 : Subsystem  Description=|  mask(Copyright Information){none=on}
      | Copyright info block.                                               
      |                                                                     
      | Place copyright information at the top of every subsystem in design.
      mask prompts: none "No parameters"
      mask help: Place copyright information at the top of every subsystem in design.
      mask Display:
      | NxtrConf = 'Nexteer Confidential';
      | 
      | sys = bdroot; %handle for the current model ("system")
      | first = get_param(sys,'Created');
      | if(isempty(first))
      |     first = datestr(now,'yyyy');
      | else
      |     first = first(end-3:end);  %year is last four digits
      | end
      | 
      | last = get_param(sys,'LastModifiedDate');
      | if isempty(last)
      |     last = datestr(now,'yyyy');
      | else
      |     last = last(end-3:end);
      | end
      | 
      | if strcmp(first,last)
      |     fprintf('%s -- Copyright %s Nexteer',NxtrConf,first)
      | else
      |     fprintf('%s -- %s%s- %s Nexteer',NxtrConf,char(169),first,last)
      | end
  Data Store Write1 : DataStoreWrite  DataStoreName=dStabyCmpNotchFil12Blnd
  Data Store Write2 : DataStoreWrite  DataStoreName=dStabyCmpNotchFil12Outp
  Data Store Write3 : DataStoreWrite  DataStoreName=dStabyCmpNotchFil1Outp
  Data Store Write4 : DataStoreWrite  DataStoreName=dStabyCmpNotchFil2Outp
  Data Store Write5 : DataStoreWrite  DataStoreName=dStabyCmpNotchFil02Blnd
  FixdToFloat_f32_u1 : FixdToFloat/FixdToFloat_f32_u16  RequirementInfo="{'linktype_rmi_doors' '0000a537 (/E-STEER Core/SubSystem Specifications/Application Functions/SF029A Stability Compensation)' '#SF029A_86' 'true' 'REQ:  SF029A_86' '' } %GIDa_c87bfa82_236a_44bd_99f0_42b17e4a2979"  Param1=14
  FixdToFloat_f32_u16 : FixdToFloat/FixdToFloat_f32_u16  RequirementInfo="{'linktype_rmi_doors' '0000a537 (/E-STEER Core/SubSystem Specifications/Application Functions/SF029A Stability Compensation)' '#SF029A_85' 'true' 'REQ:  SF029A_85' '' } %GIDa_09ff6ec6_a46d_48e1_b579_9179050fc87f"  Param1=14
  FloatToFixd_u16_f1 : FloatToFixd/FloatToFixd_u16_f32  Param1=8
  FloatToFixd_u16_f2 : FloatToFixd/FloatToFixd_u16_f32  Param1=7
  StCmp12Out : Outport
  wires:
  Blnd_f1/1 -> Blnd_f32/2  "StCmp02Out_MtrNm"
  Blnd_f32/1 -> Data Store Write2/1, StCmp12Out/1
  [VehSpd] -> BilnrIntrpnWithRound_u16_u16MplXu16MplY/2
  Compensator 1/1(Comp1_Output) -> Blnd_f32/1, Data Store Write3/1
  BilnrIntrpnWithRound_u16_u16MplXu16MplY/1 -> FixdToFloat_f32_u1/1  "CompBlnd_Uls"
  [Assist] -> Compensator 1/1(Assist)
  [Assist] -> Blnd_f1/1, Compensator 2/1(Assist)
  [HwTrqFilt] -> BilnrIntrpnWithRound_u16_u16MplXu16MplY/1
  [HwTrqFilt] -> BilnrIntrpnWithRound_u16_u16MplXu16MplY1/1
  [VehSpd] -> BilnrIntrpnWithRound_u16_u16MplXu16MplY1/2
  Compensator 2/1(Comp2_Output) -> Blnd_f1/2, Data Store Write4/1
  BilnrIntrpnWithRound_u16_u16MplXu16MplY1/1 -> FixdToFloat_f32_u16/1  "CompBlnd_Uls"
  VehSpd/1 -> FloatToFixd_u16_f2/1
  Assist/1 -> [Assist]
  HwTqFilt/1 -> FloatToFixd_u16_f1/1
  FloatToFixd_u16_f2/1 -> [VehSpd]
  FloatToFixd_u16_f1/1 -> [HwTrqFilt]
  FixdToFloat_f32_u16/1 -> Data Store Write5/1, Blnd_f1/3
  FixdToFloat_f32_u1/1 -> Data Store Write1/1, Blnd_f32/3

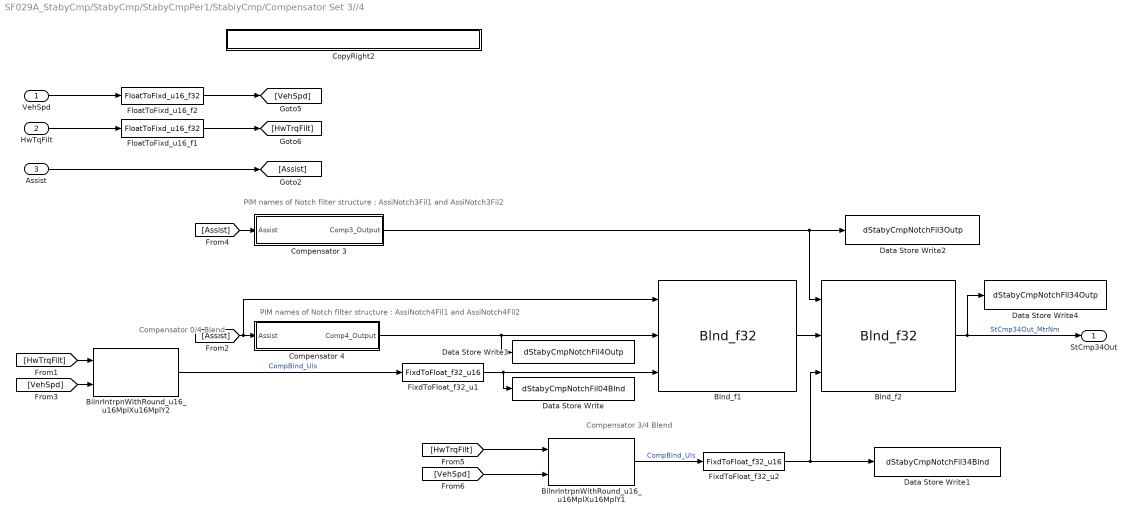
== system SF029A_StabyCmp/StabyCmp/StabyCmpPer1/StabiyCmp/Compensator Set 3//4 ==
  note: Compensator 0/4 Blend
  note: Compensator 3/4 Blend
  note: PIM names of Notch filter structure : AssiNotch3Fil1 and AssiNotch3Fil2
  note: PIM names of Notch filter structure : AssiNotch4Fil1 and AssiNotch4Fil2
  VehSpd : Inport
  HwTqFilt : Inport  Port=2
  Assist : Inport  Port=3
  BilnrIntrpnWithRound_u16_u16MplXu16MplY1 : BilnrIntrpnMplX/BilnrIntrpnWithRound_u16_u16MplXu16MplY  RequirementInfo="{'linktype_rmi_doors' '0000a537 (/E-STEER Core/SubSystem Specifications/Application Functions/SF029A Stability Compensation)' '#SF029A_91' 'true' 'REQ:  SF029A_91' '' } %GIDa_7992ea07_4f83_4ec7_855c_d2ee457ca3ac"  MplXTbl=StabyCmpNotchFilBlnd34TqX  MplYTbl=StabyCmpNotchFilBlnd34Y  BilnrSelnTbl=StabyCmpNotchFilBilnrBlndVehSpd
      settings: AttributesFormatString=|
      | Bilnr ( u16MplX , u16MplY )
      | XTbl: %<MplXTbl>
      | YTbl: %<MplYTbl>
      | BilnrSelnTbl: %<BilnrSelnTbl>
  BilnrIntrpnWithRound_u16_u16MplXu16MplY2 : BilnrIntrpnMplX/BilnrIntrpnWithRound_u16_u16MplXu16MplY  RequirementInfo="{'linktype_rmi_doors' '0000a537 (/E-STEER Core/SubSystem Specifications/Application Functions/SF029A Stability Compensation)' '#SF029A_90' 'true' 'REQ:  SF029A_90' '' } %GIDa_fa8213a5_9479_49e8_a7c2_f5e33fcb5f72"  MplXTbl=StabyCmpNotchFilBlnd34TqX  MplYTbl=StabyCmpNotchFilBlnd04Y  BilnrSelnTbl=StabyCmpNotchFilBilnrBlndVehSpd
      settings: AttributesFormatString=|
      | Bilnr ( u16MplX , u16MplY )
      | XTbl: %<MplXTbl>
      | YTbl: %<MplYTbl>
      | BilnrSelnTbl: %<BilnrSelnTbl>
  Blnd_f1 : NxtrMath/Blnd_f32  RequirementInfo="{'linktype_rmi_doors' '0000a537 (/E-STEER Core/SubSystem Specifications/Application Functions/SF029A Stability Compensation)' '#SF029A_90' 'true' 'REQ:  SF029A_90' '' } %GIDa_0c966e37_e9d2_4ab8_a8d4_bebedb6acf5c"  SFunctionSpec=single y1 = Blnd_f32(single u1, single u2, single u3)  Parameter3=on
      settings: AttributesFormatString=%<Name>
  Blnd_f2 : NxtrMath/Blnd_f32  RequirementInfo="{'linktype_rmi_doors' '0000a537 (/E-STEER Core/SubSystem Specifications/Application Functions/SF029A Stability Compensation)' '#SF029A_91' 'true' 'REQ:  SF029A_91' '' } %GIDa_c9f7afba_a480_4053_ab5f_1d5881163564"  SFunctionSpec=single y1 = Blnd_f32(single u1, single u2, single u3)  Parameter3=on
      settings: AttributesFormatString=%<Name>
  Compensator 3 : Subsystem  RequirementInfo="{'linktype_rmi_doors' '0000a537 (/E-STEER Core/SubSystem Specifications/Application Functions/SF029A Stability Compensation)' '#SF029A_89' 'true' 'REQ:  SF029A_89' '' ; 'linktype_rmi_doors' '0000a537 (/E-STEER Core/SubSystem Specifications/Application Functions/SF029A Stability Compensation)' '#SF029A_91' 'true' 'REQ:  SF029A_91' '' } %GIDa_60843c20_2c9d_458f_a1f2_2cd62789f9d9"  mask{B0=StabyCmpNotchFil3Struct.FilGainB0, B1=StabyCmpNotchFil3Struct.FilGainB1, B2=StabyCmpNotchFil3Struct.FilGainB2, A1=StabyCmpNotchFil3Struct.FilGainA1, A2=StabyCmpNotchFil3Struct.FilGainA2}
      settings: AttributesFormatString=%<Tag>
  Compensator 4 : Subsystem  RequirementInfo="{'linktype_rmi_doors' '0000a537 (/E-STEER Core/SubSystem Specifications/Application Functions/SF029A Stability Compensation)' '#SF029A_88' 'true' 'REQ:  SF029A_88' '' ; 'linktype_rmi_doors' '0000a537 (/E-STEER Core/SubSystem Specifications/Application Functions/SF029A Stability Compensation)' '#SF029A_90' 'true' 'REQ:  SF029A_90' '' } %GIDa_9ea09045_a3ce_4efb_9c3a_6b2791a6e470"  mask{B0=StabyCmpNotchFil4Struct.FilGainB0, B1=StabyCmpNotchFil4Struct.FilGainB1, B2=StabyCmpNotchFil4Struct.FilGainB2, A1=StabyCmpNotchFil4Struct.FilGainA1, A2=StabyCmpNotchFil4Struct.FilGainA2}
      settings: AttributesFormatString=%<Tag>
  CopyRight2 : Subsystem  Description=|  mask(Copyright Information){none=on}
      | Copyright info block.                                               
      |                                                                     
      | Place copyright information at the top of every subsystem in design.
      mask prompts: none "No parameters"
      mask help: Place copyright information at the top of every subsystem in design.
      mask Display:
      | NxtrConf = 'Nexteer Confidential';
      | 
      | sys = bdroot; %handle for the current model ("system")
      | first = get_param(sys,'Created');
      | if(isempty(first))
      |     first = datestr(now,'yyyy');
      | else
      |     first = first(end-3:end);  %year is last four digits
      | end
      | 
      | last = get_param(sys,'LastModifiedDate');
      | if isempty(last)
      |     last = datestr(now,'yyyy');
      | else
      |     last = last(end-3:end);
      | end
      | 
      | if strcmp(first,last)
      |     fprintf('%s -- Copyright %s Nexteer',NxtrConf,first)
      | else
      |     fprintf('%s -- %s%s- %s Nexteer',NxtrConf,char(169),first,last)
      | end
  Data Store Write : DataStoreWrite  DataStoreName=dStabyCmpNotchFil04Blnd
  Data Store Write1 : DataStoreWrite  DataStoreName=dStabyCmpNotchFil34Blnd
  Data Store Write2 : DataStoreWrite  DataStoreName=dStabyCmpNotchFil3Outp
  Data Store Write3 : DataStoreWrite  DataStoreName=dStabyCmpNotchFil4Outp
  Data Store Write4 : DataStoreWrite  DataStoreName=dStabyCmpNotchFil34Outp
  FixdToFloat_f32_u1 : FixdToFloat/FixdToFloat_f32_u16  Param1=14
  FixdToFloat_f32_u2 : FixdToFloat/FixdToFloat_f32_u16  RequirementInfo="{'linktype_rmi_doors' '0000a537 (/E-STEER Core/SubSystem Specifications/Application Functions/SF029A Stability Compensation)' '#SF029A_91' 'true' 'REQ:  SF029A_91' '' } %GIDa_30db9389_aa1e_40f7_a8f6_b80215819923"  Param1=14
  FloatToFixd_u16_f1 : FloatToFixd/FloatToFixd_u16_f32  Param1=8
  FloatToFixd_u16_f2 : FloatToFixd/FloatToFixd_u16_f32  Param1=7
  StCmp34Out : Outport
  wires:
  [VehSpd] -> BilnrIntrpnWithRound_u16_u16MplXu16MplY2/2
  [HwTrqFilt] -> BilnrIntrpnWithRound_u16_u16MplXu16MplY2/1
  [HwTrqFilt] -> BilnrIntrpnWithRound_u16_u16MplXu16MplY1/1
  [Assist] -> Blnd_f1/1, Compensator 4/1(Assist)
  [Assist] -> Compensator 3/1(Assist)
  BilnrIntrpnWithRound_u16_u16MplXu16MplY1/1 -> FixdToFloat_f32_u2/1  "CompBlnd_Uls"
  Compensator 3/1(Comp3_Output) -> Blnd_f2/1, Data Store Write2/1
  [VehSpd] -> BilnrIntrpnWithRound_u16_u16MplXu16MplY1/2
  BilnrIntrpnWithRound_u16_u16MplXu16MplY2/1 -> FixdToFloat_f32_u1/1  "CompBlnd_Uls"
  VehSpd/1 -> FloatToFixd_u16_f2/1
  Assist/1 -> [Assist]
  HwTqFilt/1 -> FloatToFixd_u16_f1/1
  Blnd_f1/1 -> Blnd_f2/2
  Blnd_f2/1 -> Data Store Write4/1, StCmp34Out/1  "StCmp34Out_MtrNm"
  FloatToFixd_u16_f1/1 -> [HwTrqFilt]
  FloatToFixd_u16_f2/1 -> [VehSpd]
  Compensator 4/1(Comp4_Output) -> Data Store Write3/1, Blnd_f1/2
  FixdToFloat_f32_u1/1 -> Data Store Write/1, Blnd_f1/3
  FixdToFloat_f32_u2/1 -> Data Store Write1/1, Blnd_f2/3

== system SF029A_StabyCmp/StabyCmp/StabyCmpPer1/StabiyCmp/CopyRight2 ==

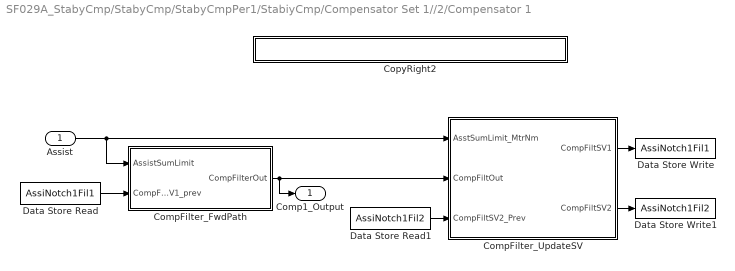
== system SF029A_StabyCmp/StabyCmp/StabyCmpPer1/StabiyCmp/Compensator Set 1//2/Compensator 1 ==
  Assist : Inport
  CompFilter_FwdPath : Subsystem
  CompFilter_UpdateSV : Subsystem
  CopyRight2 : Subsystem  Description=|  mask(Copyright Information){none=on}
      | Copyright info block.                                               
      |                                                                     
      | Place copyright information at the top of every subsystem in design.
      mask prompts: none "No parameters"
      mask help: Place copyright information at the top of every subsystem in design.
      mask Display:
      | NxtrConf = 'Nexteer Confidential';
      | 
      | sys = bdroot; %handle for the current model ("system")
      | first = get_param(sys,'Created');
      | if(isempty(first))
      |     first = datestr(now,'yyyy');
      | else
      |     first = first(end-3:end);  %year is last four digits
      | end
      | 
      | last = get_param(sys,'LastModifiedDate');
      | if isempty(last)
      |     last = datestr(now,'yyyy');
      | else
      |     last = last(end-3:end);
      | end
      | 
      | if strcmp(first,last)
      |     fprintf('%s -- Copyright %s Nexteer',NxtrConf,first)
      | else
      |     fprintf('%s -- %s%s- %s Nexteer',NxtrConf,char(169),first,last)
      | end
  Data Store Read : DataStoreRead  Priority=1  DataStoreName=AssiNotch1Fil1  DataStoreElements=AssiNotch1Fil1
  Data Store Read1 : DataStoreRead  Priority=1  DataStoreName=AssiNotch1Fil2  DataStoreElements=AssiNotch1Fil2
  Data Store Write : DataStoreWrite  Priority=2  DataStoreName=AssiNotch1Fil1  DataStoreElements=AssiNotch1Fil1
  Data Store Write1 : DataStoreWrite  Priority=2  DataStoreName=AssiNotch1Fil2  DataStoreElements=AssiNotch1Fil2
  Comp1_Output : Outport
  wires:
  CompFilter_FwdPath/1(CompFilterOut) -> Comp1_Output/1, CompFilter_UpdateSV/2(CompFiltOut)
  CompFilter_UpdateSV/1(CompFiltSV1) -> Data Store Write/1
  Data Store Read1/1 -> CompFilter_UpdateSV/3(CompFiltSV2_Prev)
  Assist/1 -> CompFilter_FwdPath/1(AssistSumLimit), CompFilter_UpdateSV/1(AsstSumLimit_MtrNm)
  Data Store Read/1 -> CompFilter_FwdPath/2(CompFiltSV1_prev)
  CompFilter_UpdateSV/2(CompFiltSV2) -> Data Store Write1/1

== system SF029A_StabyCmp/StabyCmp/StabyCmpPer1/StabiyCmp/Compensator Set 1//2/Compensator 2 ==
  Assist : Inport
  CompFilter_FwdPath : Subsystem
  CompFilter_UpdateSV : Subsystem
  CopyRight2 : Subsystem  Description=|  mask(Copyright Information){none=on}
      | Copyright info block.                                               
      |                                                                     
      | Place copyright information at the top of every subsystem in design.
      mask prompts: none "No parameters"
      mask help: Place copyright information at the top of every subsystem in design.
      mask Display:
      | NxtrConf = 'Nexteer Confidential';
      | 
      | sys = bdroot; %handle for the current model ("system")
      | first = get_param(sys,'Created');
      | if(isempty(first))
      |     first = datestr(now,'yyyy');
      | else
      |     first = first(end-3:end);  %year is last four digits
      | end
      | 
      | last = get_param(sys,'LastModifiedDate');
      | if isempty(last)
      |     last = datestr(now,'yyyy');
      | else
      |     last = last(end-3:end);
      | end
      | 
      | if strcmp(first,last)
      |     fprintf('%s -- Copyright %s Nexteer',NxtrConf,first)
      | else
      |     fprintf('%s -- %s%s- %s Nexteer',NxtrConf,char(169),first,last)
      | end
  Data Store Read : DataStoreRead  Priority=1  DataStoreName=AssiNotch2Fil1  DataStoreElements=AssiNotch2Fil1
  Data Store Read1 : DataStoreRead  Priority=1  DataStoreName=AssiNotch2Fil2  DataStoreElements=AssiNotch2Fil2
  Data Store Write : DataStoreWrite  Priority=2  DataStoreName=AssiNotch2Fil1  DataStoreElements=AssiNotch2Fil1
  Data Store Write1 : DataStoreWrite  Priority=2  DataStoreName=AssiNotch2Fil2  DataStoreElements=AssiNotch2Fil2
  Comp2_Output : Outport
  wires:
  Assist/1 -> CompFilter_UpdateSV/1(AsstSumLimit_MtrNm), CompFilter_FwdPath/1(AssistSumLimit)
  CompFilter_FwdPath/1(CompFilterOut) -> CompFilter_UpdateSV/2(CompFiltOut), Comp2_Output/1
  Data Store Read/1 -> CompFilter_FwdPath/2(CompFiltSV1_prev)
  Data Store Read1/1 -> CompFilter_UpdateSV/3(CompFiltSV2_Prev)
  CompFilter_UpdateSV/1(CompFiltSV1) -> Data Store Write/1
  CompFilter_UpdateSV/2(CompFiltSV2) -> Data Store Write1/1

== system SF029A_StabyCmp/StabyCmp/StabyCmpPer1/StabiyCmp/Compensator Set 1//2/CopyRight2 ==

== system SF029A_StabyCmp/StabyCmp/StabyCmpPer1/StabiyCmp/Compensator Set 3//4/Compensator 3 ==
  Assist : Inport
  CompFilter_FwdPath : Subsystem
  CompFilter_UpdateSV : Subsystem
  CopyRight2 : Subsystem  Description=|  mask(Copyright Information){none=on}
      | Copyright info block.                                               
      |                                                                     
      | Place copyright information at the top of every subsystem in design.
      mask prompts: none "No parameters"
      mask help: Place copyright information at the top of every subsystem in design.
      mask Display:
      | NxtrConf = 'Nexteer Confidential';
      | 
      | sys = bdroot; %handle for the current model ("system")
      | first = get_param(sys,'Created');
      | if(isempty(first))
      |     first = datestr(now,'yyyy');
      | else
      |     first = first(end-3:end);  %year is last four digits
      | end
      | 
      | last = get_param(sys,'LastModifiedDate');
      | if isempty(last)
      |     last = datestr(now,'yyyy');
      | else
      |     last = last(end-3:end);
      | end
      | 
      | if strcmp(first,last)
      |     fprintf('%s -- Copyright %s Nexteer',NxtrConf,first)
      | else
      |     fprintf('%s -- %s%s- %s Nexteer',NxtrConf,char(169),first,last)
      | end
  Data Store Read : DataStoreRead  Priority=1  DataStoreName=AssiNotch3Fil1  DataStoreElements=AssiNotch3Fil1
  Data Store Read1 : DataStoreRead  Priority=1  DataStoreName=AssiNotch3Fil2  DataStoreElements=AssiNotch3Fil2
  Data Store Write : DataStoreWrite  Priority=2  DataStoreName=AssiNotch3Fil1  DataStoreElements=AssiNotch3Fil1
  Data Store Write1 : DataStoreWrite  Priority=2  DataStoreName=AssiNotch3Fil2  DataStoreElements=AssiNotch3Fil2
  Comp3_Output : Outport
  wires:
  Assist/1 -> CompFilter_UpdateSV/1(AsstSumLimit_MtrNm), CompFilter_FwdPath/1(AssistSumLimit)
  CompFilter_FwdPath/1(CompFilterOut) -> CompFilter_UpdateSV/2(CompFiltOut), Comp3_Output/1
  Data Store Read/1 -> CompFilter_FwdPath/2(CompFiltSV1_prev)
  Data Store Read1/1 -> CompFilter_UpdateSV/3(CompFiltSV2_Prev)
  CompFilter_UpdateSV/1(CompFiltSV1) -> Data Store Write/1
  CompFilter_UpdateSV/2(CompFiltSV2) -> Data Store Write1/1
